simulink model "robotics_hover"  (R2018b)
settings: Solver=VariableStepAuto  StartTime=0.0  StopTime=25.0  RelTol=1e-3
settings Model: Creator=Shubhi  LastModifiedBy=Shubhi

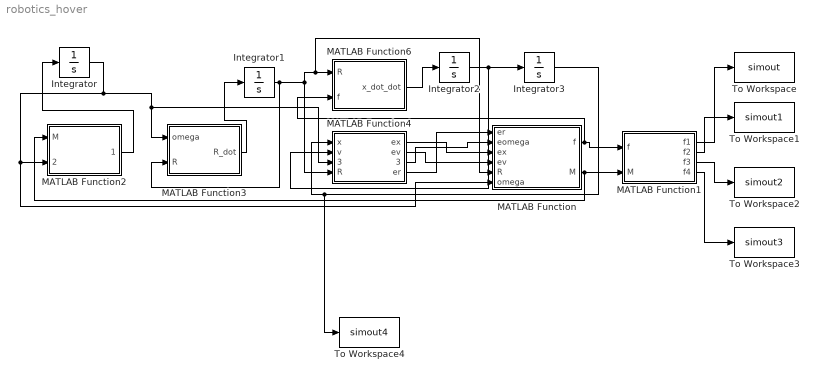
== system robotics_hover ==
  Integrator : Integrator  InitialCondition=[0;0;0]
  Integrator1 : Integrator  InitialCondition=[1,0,0;0,1,0;0,0,1]
  Integrator2 : Integrator  InitialCondition=[0;0;0]
  Integrator3 : Integrator  InitialCondition=[0;0;0]
  MATLAB Function : MATLAB Function  TreatAsAtomicUnit=on
  MATLAB Function1 : MATLAB Function  TreatAsAtomicUnit=on
  MATLAB Function2 : MATLAB Function  TreatAsAtomicUnit=on
  MATLAB Function3 : MATLAB Function  TreatAsAtomicUnit=on
  MATLAB Function4 : MATLAB Function  TreatAsAtomicUnit=on
  MATLAB Function6 : MATLAB Function  TreatAsAtomicUnit=on
  To Workspace : ToWorkspace  VariableName=simout  SaveFormat=Timeseries  SampleTime=-1
  To Workspace1 : ToWorkspace  VariableName=simout1  SaveFormat=Timeseries  SampleTime=-1
  To Workspace2 : ToWorkspace  VariableName=simout2  SaveFormat=Timeseries  SampleTime=-1
  To Workspace3 : ToWorkspace  VariableName=simout3  SaveFormat=Timeseries  SampleTime=-1
  To Workspace4 : ToWorkspace  VariableName=simout4  SaveFormat=Timeseries  SampleTime=-1
  wires:
  MATLAB Function3/1(R_dot) -> Integrator1/1
  MATLAB Function/2(M) -> MATLAB Function2/1(M), MATLAB Function1/2(M)
  Integrator/1 -> MATLAB Function4/3(omega), MATLAB Function3/1(omega), MATLAB Function/6(omega), MATLAB Function2/2(omega)
  MATLAB Function2/1(omega_dot) -> Integrator/1
  Integrator1/1 -> MATLAB Function3/2(R), MATLAB Function4/4(R), MATLAB Function/5(R), MATLAB Function6/1(R)
  MATLAB Function6/1(x_dot_dot) -> Integrator2/1
  Integrator2/1 -> MATLAB Function4/2(v), Integrator3/1
  Integrator3/1 -> To Workspace4/1, MATLAB Function4/1(x)
  MATLAB Function4/1(ex) -> MATLAB Function/3(ex)
  MATLAB Function4/2(ev) -> MATLAB Function/4(ev)
  MATLAB Function4/3(eomega) -> MATLAB Function/2(eomega)
  MATLAB Function4/4(er) -> MATLAB Function/1(er)
  MATLAB Function/1(f) -> MATLAB Function6/2(f), MATLAB Function1/1(f)
  MATLAB Function1/1(f1) -> To Workspace/1
  MATLAB Function1/2(f2) -> To Workspace1/1
  MATLAB Function1/3(f3) -> To Workspace2/1
  MATLAB Function1/4(f4) -> To Workspace3/1

== matlab function robotics_hover/MATLAB Function1 ==
  data: f input; f1 output; M input; f2 output; f3 output; f4 output
function [f1,f2,f3,f4] = fcn(f,M)


ctf=8.004*10^(-4);
d=0.315;
f4=(M(3)/ctf+f-2*M(1)/d)/4;
f2=f4+M(1)/d;
f3=(f-M(3)/(2*ctf)-f/2-M(2)/d)/2;   
f1=f3+M(2)/d;

== matlab function robotics_hover/MATLAB Function ==
  data: er input; f output; eomega input; ex input; ev input; R input; M output; omega input
function [f,M] = fcn(er,eomega,ex,ev,R,omega)
  
kx=16;
kv=5.6;
kr=8.81;
komega=2.54;

m=4.34;
g=9.8; 
e3=[0,0,1]';


f=-((-kx*ex-kv*ev-m*g*e3)')*R*e3;

Rd=[1,0,0;0,1,0;0,0,1];
omega_d=[0,0,0];

J=[0.0820,0,0;0,0.0845,0;0,0,0.1377];

M=-kr*er-komega*eomega+cross(omega,J*omega);

== matlab function robotics_hover/MATLAB Function2 ==
  data: M input; omega_dot output; omega input
function  omega_dot= fcn(M,omega)

J=[0.0820,0,0;0,0.0845,0;0,0,0.1377];
omega_dot=inv(J)*(M-cross(omega,J*omega));

== matlab function robotics_hover/MATLAB Function3 ==
  data: omega input; R_dot output; R input
function R_dot = fcn(omega,R)

 
omega_c=[0,-omega(3),omega(2);omega(3),0, -omega(1) ; -omega(2),omega(1),0];

R_dot=R*omega_c;

== matlab function robotics_hover/MATLAB Function4 ==
  data: x input; ex output; v input; omega input; R input; ev output; eomega output; er output
function [ex,ev,eomega,er] = fcn(x,v,omega,R)


ex=x-[0;0;5];
ev=v-[0;0;0];  

eomega=omega;


Rd=[1,0,0;0,1,0;0,0,1];
r =  0.5*(Rd'*R-R'*Rd);

er=[-r(2,3);r(1,3);-r(1,2)];

== matlab function robotics_hover/MATLAB Function6 ==
  data: R input; x_dot_dot output; f input
function x_dot_dot = fcn(R,f)


e3=[0;0;1];
m=4.34;
x_dot_dot=9.8*e3-(f/m)*R*e3;
